simulink model "fuc_call_inputEvent_enabling_chart_example"  (R2018a)
settings: Solver=VariableStepAuto  StartTime=0.0  StopTime=10.0  RelTol=1e-3
settings Model: Creator=86188  LastModifiedBy=86188

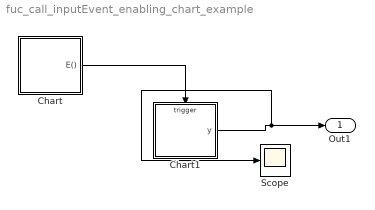
== system fuc_call_inputEvent_enabling_chart_example ==
  Chart : Stateflow chart  TreatAsAtomicUnit=on
  Chart1 : Stateflow chart  TreatAsAtomicUnit=on
  Scope : Scope
  Out1 : Outport
  wires:
  Chart/1(E()) -> Chart1/Trigger
  Chart1/1(y) -> Scope/1, Out1/1

== stateflow chart fuc_call_inputEvent_enabling_chart_example/Chart1 ==
  settings: executeAtInitialization=1
  state A
    en:y = y + 1;
    du:y = y + 1;
  (default) -> A
  data: y output double =0
  events: E input FUNCTION_CALL_EVENT

== stateflow chart fuc_call_inputEvent_enabling_chart_example/Chart ==
  state A
    bind:E;
    en:send(E);
    du:send(E);
  state B
  (default) -> A
  A -> B : after(10,tick)
  B -> A : after(10,tick)
  events: E output FUNCTION_CALL_EVENT
